simulink model "auticko"  (R2013a)
settings: Solver=ode45  StartTime=0.0  StopTime=10.0  RelTol=1e-3
settings Model: Creator=Ruddo  LastModifiedBy=Ruddo

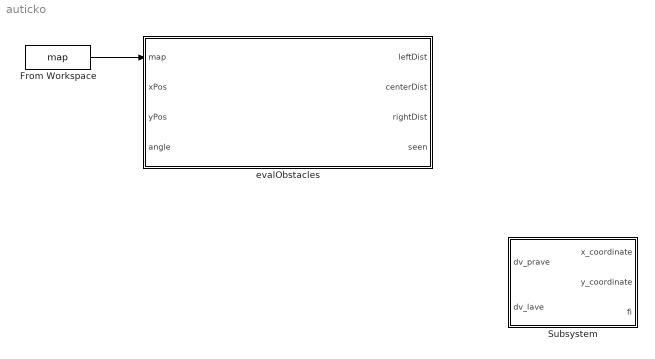
== system auticko ==
  From Workspace : FromWorkspace  VariableName=map  SampleTime=0
  Subsystem : Subsystem
  "evalObstacles " : MATLAB Function  TreatAsAtomicUnit=on
  wires:
  From Workspace/1 -> "evalObstacles "/1(map)

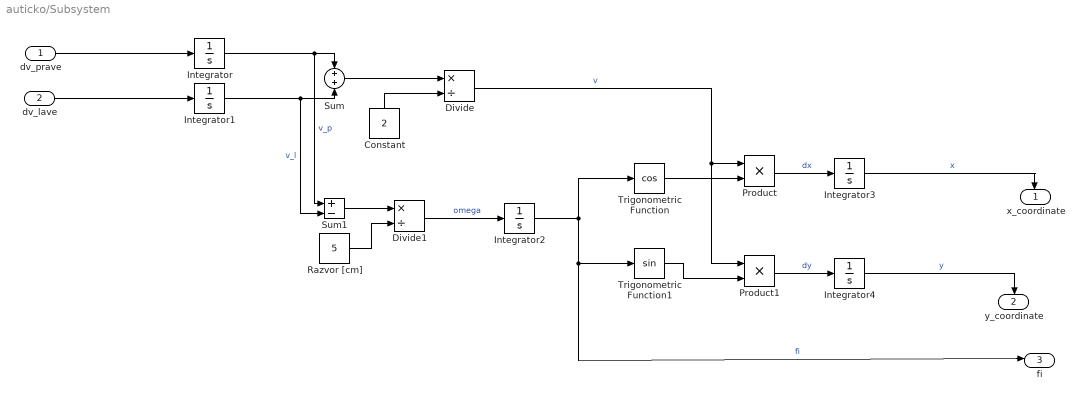
== system auticko/Subsystem ==
  dv_prave : Inport
  dv_lave : Inport  Port=2
  Constant : Constant  Value=2
  Divide : Product  Inputs=*/
  Divide1 : Product  Inputs=*/
  Integrator{,1..4} (5 alike) : Integrator
  Product : Product
  Product1 : Product
  Razvor [cm] : Constant  Value=5
  Sum : Sum
  Sum1 : Sum  Inputs=+-
  Trigonometric Function : Trigonometry  Operator=cos
  Trigonometric Function1 : Trigonometry
  x_coordinate : Outport
  y_coordinate : Outport  Port=2
  "fi " : Outport  Port=3
  wires:
  Divide/1 -> Product/1, Product1/1  "v"
  Integrator1/1 -> Sum1/2, Sum/2  "v_l"
  Integrator/1 -> Sum1/1, Sum/1  "v_p"
  Constant/1 -> Divide/2
  Trigonometric Function/1 -> Product/2
  Integrator2/1 -> "fi "/1, Trigonometric Function1/1, Trigonometric Function/1  "fi"
  Product1/1 -> Integrator4/1  "dy"
  Sum/1 -> Divide/1
  Product/1 -> Integrator3/1  "dx"
  Trigonometric Function1/1 -> Product1/2
  dv_prave/1 -> Integrator/1
  Integrator3/1 -> x_coordinate/1  "x"
  dv_lave/1 -> Integrator1/1
  Sum1/1 -> Divide1/1
  Divide1/1 -> Integrator2/1  "omega"
  Razvor [cm]/1 -> Divide1/2
  Integrator4/1 -> y_coordinate/1  "y"

== matlab function auticko/evalObstacles  ==
  data: map input; leftDist output; xPos input; yPos input; angle input; centerDist output; rightDist output; seen output
%vseobecne pre mapu m x n
%vyhodnoti co vidia ultrazvuky
%vracia vzdialenost v akej vidi pravy, sredny a lavy sonar prekazku. Dosah = pol metra = 5 policok
%Vzdy vracia na kazdom senzore iba najblizsiu prekazku
%
%dist = 9999 -> dany senzor nevidi prekazku
%rozsahy oproti natoceniu robota:
%lavy ultrazvuk:        +45 - +15 stupnov
%stredny ultrazvuk:     +15 - -15 stupnov
%pravy ultrazvuk:       -15 - -45 stupnov
%
%
%map - mapa (mriezka m x n) v mierke 1:10 
%xPos -xova suradnica robota
%yPos - ylonova suradnica robota
%uhol natocenia robota - 0 stupnov = doprava

function [leftDist,centerDist,rightDist,seen] = evalObstacles(map,xPos,yPos,angle )
    seen=[];
    leftDist = 9999;
    centerDist = 9999;
    rightDist = 9999;
    [rows,columns] = size(map);

    xFrom = round(xPos/10)-6;
    yFrom = round(yPos/10)-6;
    xTo = round(xPos/10)+6;
    yTo = round(yPos/10)+6;

    if (xFrom <1)
        xFrom =1;
    end;

    if (yFrom <1)
        yFrom =1;
    end;

    if (xTo>columns )
        xTo =columns;
    end;

    if (yTo > rows)
        yTo = rows;
    end;
    
    for x = xFrom:1:xTo
        for y = yFrom:1:yTo
            if (map(x,y) == 1)
                dx = xPos-10*x;
                dy = yPos-10*y;
                
                modif =0;
                if 10*x > xPos && 10*y>yPos        %I. kvadrant
                    modif = 0;
                end;
                if 10*x < xPos && 10*y > yPos      %II. kvadrant
                    modif=90;        
                end;
                if 10*x < xPos && 10*y < yPos      %III. kvadrant
                    modif=180;
                end;
                if 10*x > xPos && 10*y < yPos      %IV. kvadrant
                    modif = 270;
                end;
                
                
                obstacleAngle = rad2deg(asin(abs(dy)/sqrt(dx^2+dy^2)))+modif; % uhol prekazky voci osi x od auticka
                
                %zorny uhol pod ktorym auticko vidi prekazku
                visDiff = angle-obstacleAngle;
                %visDiff = visAngle-angle;
                
                obstDist = sqrt(dx^2+dy^2);
                obstSeen=0;
                
                if (obstDist < 50)
                    %pravy
                    if (45 >= visDiff && visDiff >15)
                        if (obstDist <rightDist )
                            rightDist = obstDist;
                            
                        end;
                         obstSeen=1;
                    end; 

                    %stredny
                    if (15 >= visDiff && visDiff > -15)
                        if (obstDist <centerDist )
                            centerDist = obstDist;
                        end;
                         obstSeen=1;
                    end;

                    %lavy
                    if (-15 >= visDiff && visDiff >= -45)
                        if (obstDist <leftDist )
                            leftDist = obstDist;
                        end;
                        obstSeen=1;
                    end;
                
                    if (obstSeen ==1)
                        [xPos,yPos,x*10,y*10,angle,obstacleAngle,visDiff];
                        [r,c] = size(seen);
                        seen(1,c+1) = x;
                        seen(2,c+1) = y;
                    end;
                    
                end;
            end;
        end;
    end;
end
